simulink model "washout_filter_sim"  (R2022b)
settings: Solver=VariableStepAuto  StartTime=9.99  StopTime=37.23  RelTol=1e-3
values from neighbouring files (symbols this model uses):
  Cf = 200000    [Init_for_washout_filter.m]    (also in UKF_start.m)
  Cr = 250000    [Init_for_washout_filter.m]    (also in UKF_start.m)
  lf = 1.65    [Init_for_washout_filter.m]    (also in UKF_start.m)
  lr = L-lf    (= 1.291)    [Init_for_washout_filter.m]    (also in UKF_start.m)
  mass = 2010.5    [Init_for_washout_filter.m]    (also in UKF_start.m)
  Ratio = 16.3    [Init_for_washout_filter.m]    (also in UKF_start.m)
  rollGrad = 4.5    [Init_for_washout_filter.m]    (also in UKF_start.m)
  rx = 0.29    [Init_for_washout_filter.m]    (also in UKF_start.m)
  ry = 0    [Init_for_washout_filter.m]    (also in UKF_start.m)
  T = 0.01    [Init_for_washout_filter.m]
  Ts = 0.01    [Init_for_washout_filter.m]    (also in UKF_start.m)
undefined symbols (not defined in the file or in its folder): a, b, c
libraries: hdlsllib x1, simulink_extras x1
settings Model: Creator=tawsi_000  LastModifiedBy=tawsi_000

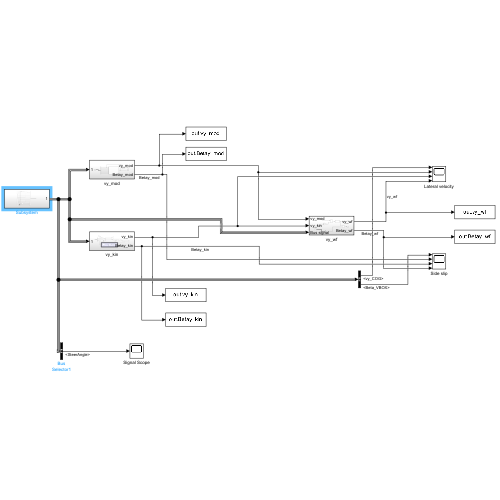
[thumbnail: Simulink's stored preview of the top-level diagram]
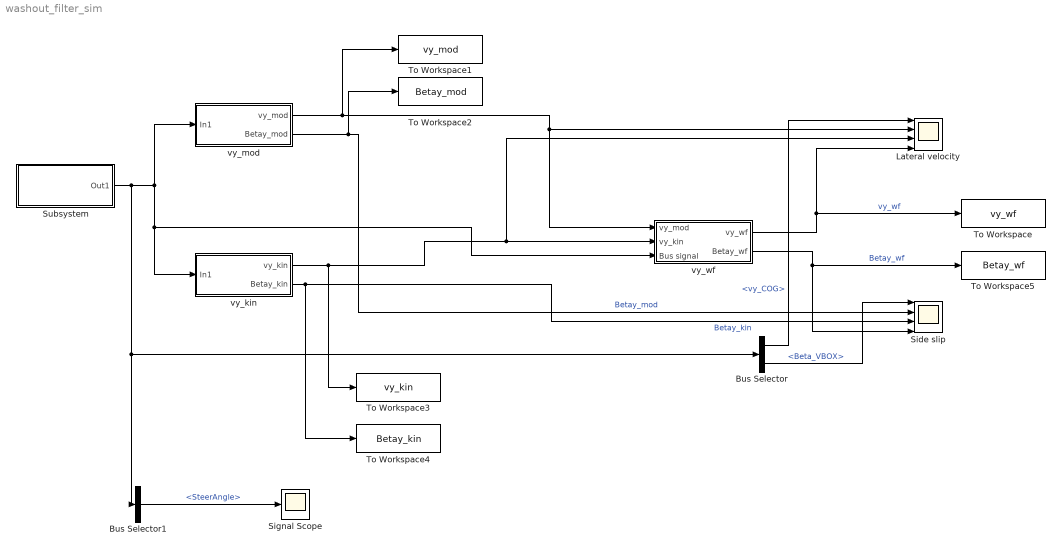
== system washout_filter_sim ==
  Bus Selector : BusSelector  OutputSignals=vy_COG,Beta_VBOX
  Bus Selector1 : BusSelector  OutputSignals=SteerAngle
  Lateral velocity : Scope  NumInputPorts=4
  Side slip : Scope  NumInputPorts=4
  Signal Scope : Scope
  Subsystem : Subsystem
  To Workspace : ToWorkspace  VariableName=vy_wf  SaveFormat=Timeseries  SampleTime=-1
  To Workspace1 : ToWorkspace  VariableName=vy_mod  SaveFormat=Timeseries  SampleTime=-1
  To Workspace2 : ToWorkspace  VariableName=Betay_mod  SaveFormat=Timeseries  SampleTime=-1
  To Workspace3 : ToWorkspace  VariableName=vy_kin  SaveFormat=Timeseries  SampleTime=-1
  To Workspace4 : ToWorkspace  VariableName=Betay_kin  SaveFormat=Timeseries  SampleTime=-1
  To Workspace5 : ToWorkspace  VariableName=Betay_wf  SaveFormat=Timeseries  SampleTime=-1
  vy_kin : Subsystem
  vy_mod : Subsystem
  vy_wf : Subsystem
  wires:
  vy_wf/1(vy_wf) -> Lateral velocity/4, To Workspace/1  "vy_wf"
  Subsystem/1(Out1) -> Bus Selector1/1, Bus Selector/1, vy_kin/1(In1), vy_wf/3(Bus signal), vy_mod/1(In1)
  vy_mod/2(Betay_mod) -> To Workspace2/1, Side slip/2  "Betay_mod"
  vy_kin/2(Betay_kin) -> To Workspace4/1, Side slip/3  "Betay_kin"
  vy_mod/1(vy_mod) -> To Workspace1/1, Lateral velocity/2, vy_wf/1(vy_mod)
  vy_kin/1(vy_kin) -> To Workspace3/1, Lateral velocity/3, vy_wf/2(vy_kin)
  vy_wf/2(Betay_wf) -> To Workspace5/1, Side slip/4  "Betay_wf"
  Bus Selector/2 -> Side slip/1  "<Beta_VBOX>"
  Bus Selector/1 -> Lateral velocity/1  "<vy_COG>"
  Bus Selector1/1 -> Signal Scope/1  "<SteerAngle>"

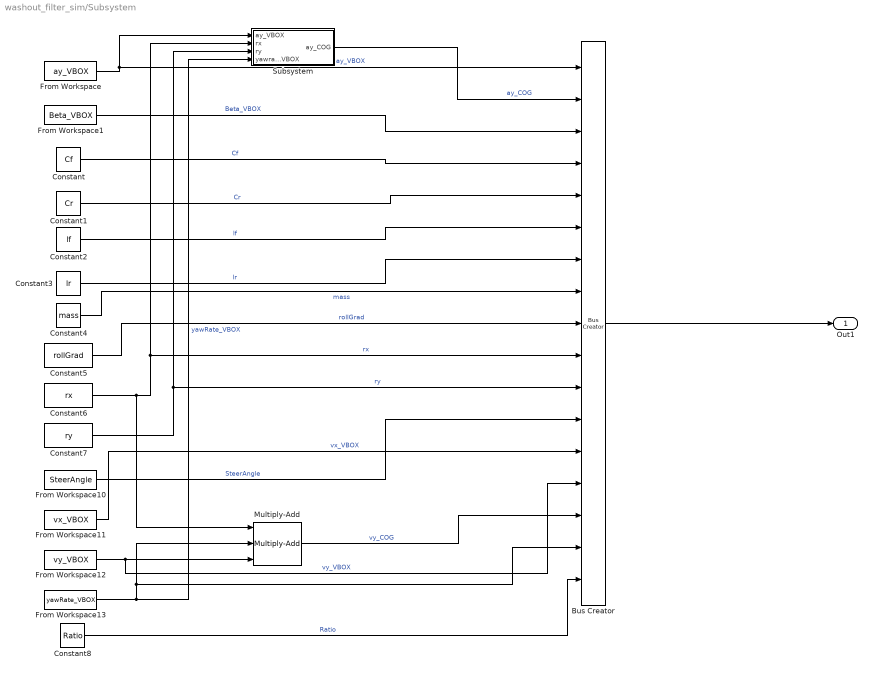
== system washout_filter_sim/Subsystem ==
  Bus Creator : BusCreator  Inputs=17
  Constant : Constant  Value=Cf
  Constant1 : Constant  Value=Cr
  Constant2 : Constant  Value=lf
  Constant3 : Constant  Value=lr
  Constant4 : Constant  Value=mass
  Constant5 : Constant  Value=rollGrad
  Constant6 : Constant  Value=rx
  Constant7 : Constant  Value=ry
  Constant8 : Constant  Value=Ratio
  From Workspace : FromWorkspace  VariableName=ay_VBOX  SampleTime=Ts
  From Workspace1 : FromWorkspace  VariableName=Beta_VBOX  SampleTime=Ts
  From Workspace10 : FromWorkspace  VariableName=SteerAngle  SampleTime=Ts
  From Workspace11 : FromWorkspace  VariableName=vx_VBOX  SampleTime=Ts
  From Workspace12 : FromWorkspace  VariableName=vy_VBOX  SampleTime=Ts
  From Workspace13 : FromWorkspace  VariableName=yawRate_VBOX  SampleTime=Ts
  Multiply-Add : hdlsllib/HDL Operations/Multiply-Add  Function=c+(a.*b)  datatype=Inherit: Inherit via internal rule  DoSatur=off  FMA=off
  Subsystem : Subsystem
  Out1 : Outport
  wires:
  From Workspace/1 -> Subsystem/1(ay_VBOX), Bus Creator/1  "ay_VBOX"
  From Workspace1/1 -> Bus Creator/3  "Beta_VBOX"
  Constant/1 -> Bus Creator/4  "Cf"
  Constant1/1 -> Bus Creator/5  "Cr"
  Constant2/1 -> Bus Creator/6  "lf"
  Constant3/1 -> Bus Creator/7  "lr"
  Bus Creator/1 -> Out1/1
  Constant4/1 -> Bus Creator/8  "mass"
  Constant5/1 -> Bus Creator/9  "rollGrad"
  From Workspace12/1 -> Multiply-Add/3, Bus Creator/14  "vy_VBOX"
  Constant6/1 -> Subsystem/2(rx), Bus Creator/10, Multiply-Add/1  "rx"
  From Workspace13/1 -> Subsystem/4(yawrate_VBOX), Multiply-Add/2, Bus Creator/16  "yawRate_VBOX"
  Constant7/1 -> Subsystem/3(ry), Bus Creator/11  "ry"
  From Workspace10/1 -> Bus Creator/12  "SteerAngle"
  From Workspace11/1 -> Bus Creator/13  "vx_VBOX"
  Multiply-Add/1 -> Bus Creator/15  "vy_COG"
  Subsystem/1(ay_COG) -> Bus Creator/2  "ay_COG"
  Constant8/1 -> Bus Creator/17  "Ratio"

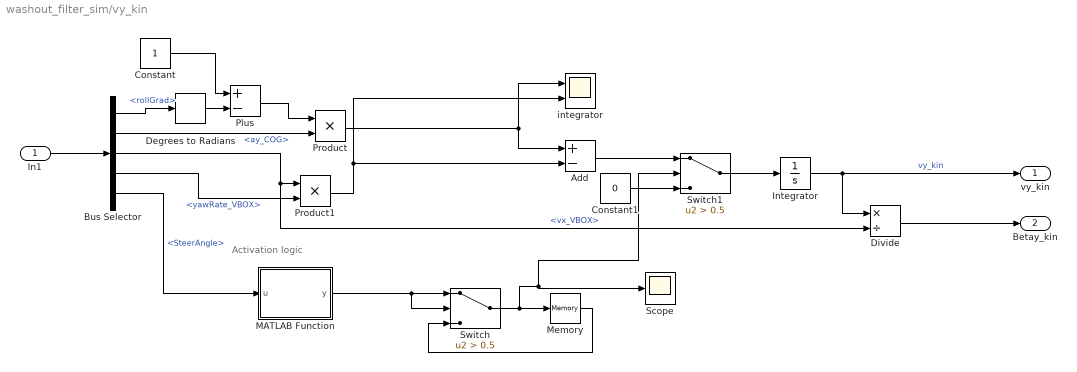
== system washout_filter_sim/vy_kin ==
  note: Activation logic
  In1 : Inport
  Add : Sum  Inputs=+-
  Bus Selector : BusSelector  OutputSignals=rollGrad,ay_COG,vx_VBOX,yawRate_VBOX,SteerAngle
  Constant : Constant
  Constant1 : Constant  Value=0
  Degrees to Radians : simulink_extras/Transformations/Degrees to Radians
  Divide : Product  Inputs=*/
  Integrator : Integrator
  MATLAB Function : MATLAB Function  TreatAsAtomicUnit=on
  Memory : Memory
  Plus : Sum  Inputs=+-
  Product : Product
  Product1 : Product
  Scope : Scope
  Switch : Switch  Criteria=u2 > Threshold  Threshold=0.5  SaturateOnIntegerOverflow=off  InputSameDT=off
  Switch1 : Switch  Criteria=u2 > Threshold  Threshold=0.5  SaturateOnIntegerOverflow=off  InputSameDT=off
  integrator : Scope  NumInputPorts=2
  vy_kin : Outport
  Betay_kin : Outport  Port=2
  wires:
  Bus Selector/5 -> MATLAB Function/1(u)  "<SteerAngle>"
  Bus Selector/4 -> Product1/2  "<yawRate_VBOX>"
  MATLAB Function/1(y) -> Switch/2, Switch/1
  Product/1 -> integrator/1, Add/1
  Bus Selector/2 -> Product/2  "<ay_COG>"
  Constant/1 -> Plus/1
  Divide/1 -> Betay_kin/1
  Degrees to Radians/1 -> Plus/2
  Bus Selector/3 -> Divide/2, Product1/1  "<vx_VBOX>"
  Plus/1 -> Product/1
  Memory/1 -> Switch/3
  Bus Selector/1 -> Degrees to Radians/1  "<rollGrad>"
  Product1/1 -> Add/2, integrator/2
  Switch/1 -> Switch1/2, Scope/1, Memory/1
  Add/1 -> Switch1/1
  Integrator/1 -> vy_kin/1, Divide/1  "vy_kin"
  In1/1 -> Bus Selector/1
  Constant1/1 -> Switch1/3
  Switch1/1 -> Integrator/1

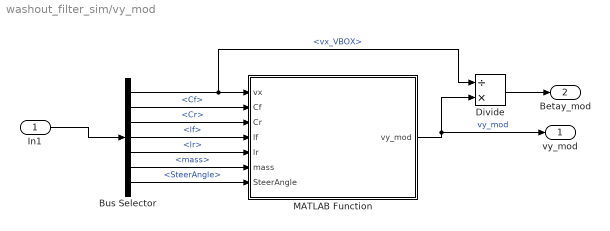
== system washout_filter_sim/vy_mod ==
  In1 : Inport
  Bus Selector : BusSelector  OutputSignals=vx_VBOX,Cf,Cr,lf,lr,mass,SteerAngle
  Divide : Product  Inputs=/*
  MATLAB Function : MATLAB Function  TreatAsAtomicUnit=on
  vy_mod : Outport
  Betay_mod : Outport  Port=2
  wires:
  In1/1 -> Bus Selector/1
  Bus Selector/1 -> Divide/1, MATLAB Function/1(vx)  "<vx_VBOX>"
  Bus Selector/2 -> MATLAB Function/2(Cf)  "<Cf>"
  Bus Selector/3 -> MATLAB Function/3(Cr)  "<Cr>"
  Bus Selector/4 -> MATLAB Function/4(lf)  "<lf>"
  Bus Selector/5 -> MATLAB Function/5(lr)  "<lr>"
  Bus Selector/6 -> MATLAB Function/6(mass)  "<mass>"
  Bus Selector/7 -> MATLAB Function/7(SteerAngle)  "<SteerAngle>"
  MATLAB Function/1(vy_mod) -> Divide/2, vy_mod/1  "vy_mod"
  Divide/1 -> Betay_mod/1

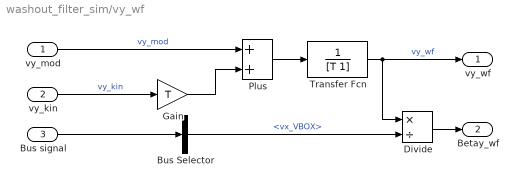
== system washout_filter_sim/vy_wf ==
  vy_mod : Inport
  vy_kin : Inport  Port=2
  Bus signal : Inport  Port=3
  Bus Selector : BusSelector  OutputSignals=vx_VBOX
  Divide : Product  Inputs=*/
  Gain : Gain  Gain=T
  Plus : Sum
  Transfer Fcn : TransferFcn  Denominator=[T 1]
  vy_wf : Outport
  Betay_wf : Outport  Port=2
  wires:
  Gain/1 -> Plus/2
  vy_mod/1 -> Plus/1  "vy_mod"
  vy_kin/1 -> Gain/1  "vy_kin"
  Plus/1 -> Transfer Fcn/1
  Transfer Fcn/1 -> Divide/1, vy_wf/1  "vy_wf"
  Bus signal/1 -> Bus Selector/1
  Bus Selector/1 -> Divide/2  "<vx_VBOX>"
  Divide/1 -> Betay_wf/1

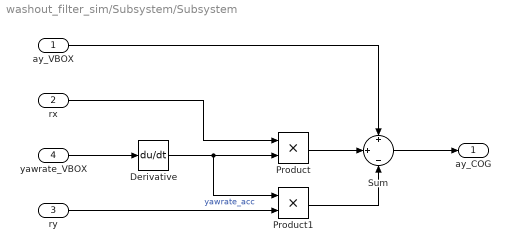
== system washout_filter_sim/Subsystem/Subsystem ==
  ay_VBOX : Inport
  rx : Inport  Port=2
  ry : Inport  Port=3
  yawrate_VBOX : Inport  Port=4
  Derivative : Derivative
  Product : Product
  Product1 : Product
  Sum : Sum  Inputs=+|+|-
  ay_COG : Outport
  wires:
  yawrate_VBOX/1 -> Derivative/1
  Derivative/1 -> Product1/1, Product/2  "yawrate_acc"
  rx/1 -> Product/1
  ry/1 -> Product1/2
  Product/1 -> Sum/2
  ay_VBOX/1 -> Sum/1
  Product1/1 -> Sum/3
  Sum/1 -> ay_COG/1

== matlab function washout_filter_sim/vy_kin/MATLAB Function ==
  data: u input; y output
function y = fcn(u)

if abs(u)>0.03
    y=1;
else
    y=0;
end

== matlab function washout_filter_sim/vy_mod/MATLAB Function ==
  data: vx input; vy_mod output; Cf input; Cr input; lf input; lr input; mass input; SteerAngle input
function vy_mod = fcn(vx, Cf, Cr, lf, lr, mass, SteerAngle)

vy_mod = SteerAngle*(vx*(lr*Cf*Cr*(lf+lr)-lf*Cf*mass*(vx.^2)))...
    /((lf+lr)^2*Cf*Cr+mass*(vx^2)*(lr*Cr-lf*Cf));
